simulink model "QuarcCLVI"  (R2019a)
settings: Solver=FixedStepDiscrete  StartTime=0.0  StopTime=inf  FixedStep=0.03  RelTol=1e-3  EnableMultiTasking=on
undefined symbols (not defined in the file): qc_get_step_size
libraries: quarc_library x5, cstblocks x1, simulink_extras x1
settings Model: SimulationMode=external  ExtModeTrigDuration=10000  Creator=alberto.cruz6  LastModifiedBy=marcos.pesante
settings SolverCC: PositivePriorityOrder=on
settings RTWCC: SystemTargetFile=quarc_win64.tlc  TemplateMakefile=quarc_default_tmf  Description=QUARC Win64 Target
settings STFCustomTargetCC: TargetPreCompLibLocation=C:\PROGRA~3\QUARC\lib\2019a\win64\release  TargetLangStandard=C99 (ISO)  ConcurrentExecutionCompliant=on  SystemTargetFile=quarc_win64.tlc
settings GRTTargetCC: TargetPreCompLibLocation=C:\PROGRA~3\QUARC\lib\2019a\win64\release  ParMdlRefBuildCompliant=off  CompOptLevelCompliant=off  CombineOutputUpdateFcns=off  MatFileLogging=off  CPPClassGenCompliant=off  GRTInterface=on  UseToolchainInfoCompliant=off  ExtMode=on  ExtModeMexFile=quarc_comm

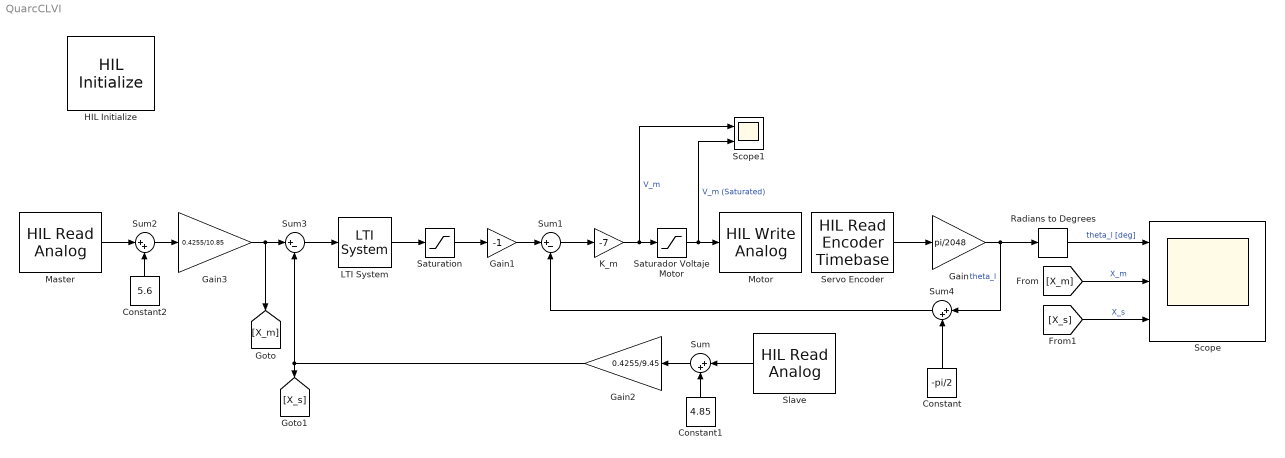
== system QuarcCLVI ==
  Constant : Constant  Value=-pi/2
  Constant1 : Constant  Value=4.85
  Constant2 : Constant  Value=5.6
  Gain : Gain  Gain=pi/2048
  Gain1 : Gain  Gain=-1
  Gain2 : Gain  Gain=0.4255/9.45
  Gain3 : Gain  Gain=0.4255/10.85
  HIL Initialize : quarc_library/Data Acquisition/Generic/Configuration/HIL Initialize  object_name=DAQ  board_type=q8_usb  board_number=0  board_options=update_rate=normal;decimation=1  exclusive=off  active=on  hardware_clocks=[0:2]  clock_modes=[]  initial_clock_frequencies=[]  set_clock_params_at_start=off  set_clock_params_at_switch_in=off  set_clock_frequencies_at_start=off  set_clock_frequencies_at_switch_in=off  analog_input_channels=[0:7]  analog_input_configurations=[]  analog_input_maximums=10  analog_input_minimums=-10  set_analog_input_params_at_start=on  set_analog_input_params_at_switch_in=off  analog_output_channels=[0:7]  analog_output_maximums=10  analog_output_minimums=-10  initial_analog_outputs=[0]  final_analog_outputs=[0]  watchdog_analog_outputs=0  set_analog_output_params_at_start=on  set_analog_output_params_at_switch_in=off  set_analog_outputs_at_start=on  set_analog_outputs_at_switch_in=off  set_analog_outputs_at_terminate=on  set_analog_outputs_at_switch_out=off  set_analog_outputs_on_watchdog=off  digital_input_channels=[]  digital_output_channels=[]  digital_output_configuration=[]  initial_digital_outputs=[1]  final_digital_outputs=[1]  watchdog_digital_outputs=[1]  set_digital_output_params_at_start=off  set_digital_output_params_at_switch_in=off  set_digital_outputs_at_start=on  set_digital_outputs_at_switch_in=off  set_digital_outputs_at_terminate=on  set_digital_outputs_at_switch_out=off  set_digital_outputs_on_watchdog=off  encoder_channels=[0:7]  quadrature=[4]  encoder_filter_frequency=[]  initial_encoder_counts=[0]  set_encoder_params_at_start=on  set_encoder_params_at_switch_in=off  set_encoder_counts_at_start=on  set_encoder_counts_at_switch_in=off  pwm_channels=[0:7]  pwm_modes=0  pwm_frequency=99.532799999999995e6/4095  pwm_configuration=[0]  pwm_alignment=[0]  pwm_polarity=[1]  pwm_leading_deadband=[0]  pwm_trailing_deadband=[0]  initial_pwm_outputs=[0]  final_pwm_outputs=[0]  watchdog_pwm_outputs=[0]  set_pwm_params_at_start=on  set_pwm_params_at_switch_in=off  set_pwm_outputs_at_start=on  set_pwm_outputs_at_switch_in=off  set_pwm_outputs_at_terminate=on  set_pwm_outputs_at_switch_out=off  set_pwm_outputs_on_watchdog=off  other_output_channels=[]  initial_other_outputs=[]  final_other_outputs=[]  watchdog_other_outputs=[]  set_other_outputs_at_start=off  set_other_outputs_at_switch_in=off  set_other_outputs_at_terminate=off  set_other_outputs_at_switch_out=off  set_other_outputs_on_watchdog=off
  "K_m " : Gain  Gain=-7
  LTI System : cstblocks/LTI System  sys=G_c  IC=[]
  Master : quarc_library/Data Acquisition/Generic/Immediate I//O/HIL Read Analog  object_name=DAQ  channels=[1]  sample_time=qc_get_step_size  active=on  vector_output=off
  Motor : quarc_library/Data Acquisition/Generic/Immediate I//O/HIL Write Analog  object_name=DAQ  channels=0  sample_time=-1  active=off  vector_input=off
  Radians to Degrees : simulink_extras/Transformations/Radians to Degrees
  Saturador Voltaje Motor : Saturate  UpperLimit=5  LowerLimit=-5
  Saturation : Saturate  UpperLimit=pi/2  LowerLimit=-pi/2
  Scope : Scope  NumInputPorts=3
  Scope1 : Scope  NumInputPorts=2
  Servo Encoder : quarc_library/Data Acquisition/Generic/Timebases/HIL Read Encoder Timebase  object_name=DAQ  clock=0  channels=0  samples_in_buffer=max(ceil(1/qc_get_step_size), 1)  active=on  vector_output=off  data_type_mode=Inherit via back propagation  data_type=double
  Slave : quarc_library/Data Acquisition/Generic/Immediate I//O/HIL Read Analog  object_name=DAQ  channels=[0]  sample_time=qc_get_step_size  active=on  vector_output=off
  Sum : Sum  Inputs=|++
  Sum1 : Sum  Inputs=|+-
  Sum2 : Sum  Inputs=|++
  Sum3 : Sum  Inputs=|+-
  Sum4 : Sum  Inputs=|++
  wires:
  Saturador Voltaje Motor/1 -> Scope1/2, Motor/1  "V_m (Saturated)"
  Sum1/1 -> "K_m "/1
  Servo Encoder/1 -> Gain/1
  "K_m "/1 -> Scope1/1, Saturador Voltaje Motor/1  "V_m"
  Gain/1 -> Sum4/1, Radians to Degrees/1  "theta_l"
  Gain2/1 -> [X_s], Sum3/2
  Radians to Degrees/1 -> Scope/1  "theta_l [deg]"
  LTI System/1 -> Saturation/1
  Saturation/1 -> Gain1/1
  Sum3/1 -> LTI System/1
  Sum2/1 -> Gain3/1
  Constant2/1 -> Sum2/2
  Master/1 -> Sum2/1
  Gain3/1 -> [X_m], Sum3/1
  Sum/1 -> Gain2/1
  Constant1/1 -> Sum/2
  Slave/1 -> Sum/1
  Gain1/1 -> Sum1/1
  Sum4/1 -> Sum1/2
  Constant/1 -> Sum4/2
  [X_m] -> Scope/2  "X_m"
  [X_s] -> Scope/3  "X_s"
